simulink subsystem "Wind_and_Turbulence"  (R2024b)
settings: Solver=VariableStepAuto  StartTime=0.0  StopTime=10.0  RelTol=1e-3
undefined symbols (not defined in the file): F, MIL, turbulence_noise_seeds
libraries: aerolibwind2 x1
settings Model: Creator=thatf  LastModifiedBy=thatf

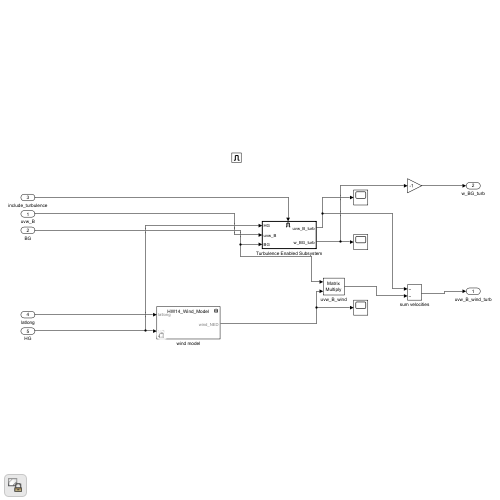
[thumbnail: Simulink's stored preview of the top-level diagram]
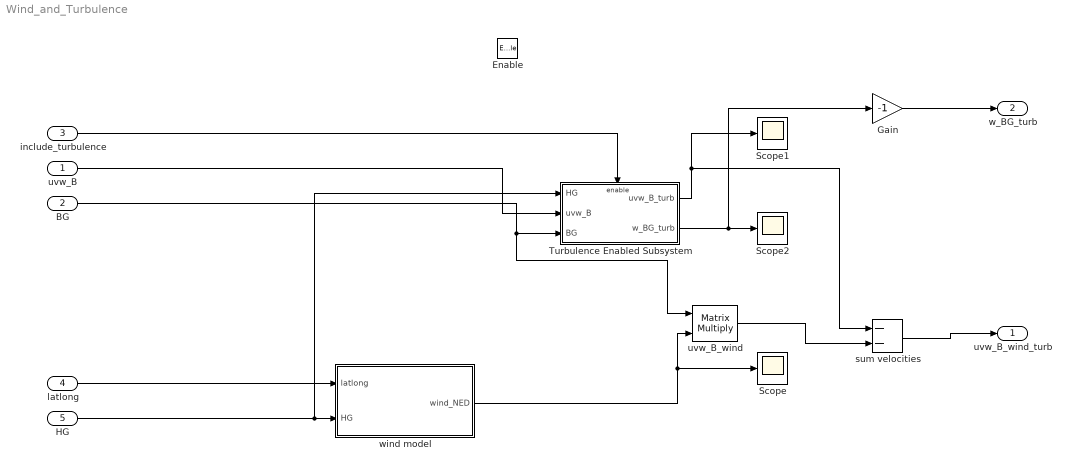
== system Wind_and_Turbulence ==
  uvw_B : Inport
  BG : Inport  Port=2
  include_turbulence : Inport  Port=3
  latlong : Inport  Port=4
  HG : Inport  Port=5
  Enable : EnablePort
  Gain : Gain  Gain=-1
  Scope : Scope
  Scope1 : Scope
  Scope2 : Scope
  Turbulence Enabled Subsystem : Subsystem  TreatAsAtomicUnit=on
  sum velocities : Sum  Inputs=--
  uvw_B_wind : Product  Multiplication=Matrix(*)
  wind model : Subsystem  Variant=on  VariantChoicesSpecifier={'Wind_Model_Systems/*.slx'}  VariantChoicesEnumeration=WindModelType  VariantControlVariable=wind_model_type
  uvw_B_wind_turb : Outport
  w_BG_turb : Outport  Port=2
  wires:
  BG/1 -> Turbulence Enabled Subsystem/3(BG), uvw_B_wind/1
  Gain/1 -> w_BG_turb/1
  HG/1 -> Turbulence Enabled Subsystem/1(HG), wind model/2(HG)
  uvw_B/1 -> Turbulence Enabled Subsystem/2(uvw_B)
  wind model/1(wind_NED) -> Scope/1, uvw_B_wind/2
  latlong/1 -> wind model/1(latlong)
  uvw_B_wind/1 -> sum velocities/2
  sum velocities/1 -> uvw_B_wind_turb/1
  include_turbulence/1 -> Turbulence Enabled Subsystem/Enable
  Turbulence Enabled Subsystem/2(w_BG_turb) -> Scope2/1, Gain/1
  Turbulence Enabled Subsystem/1(uvw_B_turb) -> sum velocities/1, Scope1/1

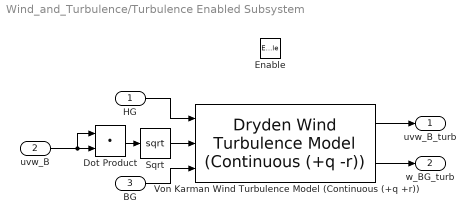
== system Wind_and_Turbulence/Turbulence Enabled Subsystem ==
  HG : Inport
  uvw_B : Inport  Port=2
  BG : Inport  Port=3
  Enable : EnablePort
  Dot Product : DotProduct  OutDataTypeStr=Inherit: Inherit via internal rule
  Sqrt : Sqrt
  Von Karman Wind Turbulence Model (Continuous (+q +r)) : aerolibwind2/Dryden Wind Turbulence Model  (Continuous (+q -r))  units=Metric (MKS)  spec=MIL-F-8785C  model=Continuous Von Karman (+q +r)  W20=wind_speed6m  Wdeg=wind_direction6m  TurbProb=10^-1  L_high=762  Wingspan=finspan  ts=0.1  Seed=turbulence_noise_seeds  T_on=on
  uvw_B_turb : Outport
  w_BG_turb : Outport  Port=2
  wires:
  Von Karman Wind Turbulence Model (Continuous (+q +r))/2 -> w_BG_turb/1
  HG/1 -> Von Karman Wind Turbulence Model (Continuous (+q +r))/1
  Von Karman Wind Turbulence Model (Continuous (+q +r))/1 -> uvw_B_turb/1
  BG/1 -> Von Karman Wind Turbulence Model (Continuous (+q +r))/3
  Dot Product/1 -> Sqrt/1
  uvw_B/1 -> Dot Product/2, Dot Product/1
  Sqrt/1 -> Von Karman Wind Turbulence Model (Continuous (+q +r))/2

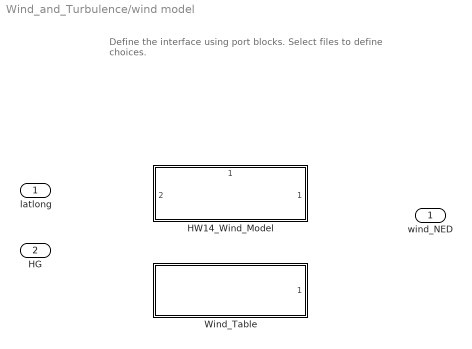
== system Wind_and_Turbulence/wind model ==
  note: Define the interface using port blocks.
      | Select files to define choices.
  latlong : Inport
  HG : Inport  Port=2
  HW14_Wind_Model : Subsystem  VariantControl=wind_model_type == WindModelType.HW14_Wind_Model  ReferencedSubsystem=HW14_Wind_Model
      settings: PortSchema="{\"entries\":[{\"content\":{\"sides\":[{\"content\":{\"connectorIds\":[\"In2\"]},\"type\":\"ConnectorPlacement.EquallySpacedRectSide\",\"uuid\":\"d8bf0063-a5dc-4cdf-b0cd-a42a4ee08dc2\"},{\"content\":{\"connectorIds\":[\"Out1\"],\"side\":\"RIGHT\"},\"type\":\"ConnectorPlacement.EquallySpacedRectSide\",\"uuid\":\"34066ee5-a4bd-4bc0-8f39-e852a60891f7\"},{\"content\":{\"connectorIds\":[\"In1\"],\"side\":\"TOP\"},\"type\":\"ConnectorPlacement.EquallySpacedRectSide\",\"uuid\":\"a97e4526-6fd6-4600-b083-aa766868201e\"}]},\"type\":\"ConnectorPlacement.EquallySpacedConnector\",\"uuid\":\"137278df-0248-4679-a789-a3816a186ef9\"}],\"packageUris\":[\"http://schema.mathworks.com/mf0/Connector/R2020b\"],\"version\":\"1.0\"}"
  Wind_Table : Subsystem  VariantControl=wind_model_type == WindModelType.Wind_Table  ReferencedSubsystem=Wind_Table
  wind_NED : Outport
